simulink model "Day1"  (R2021a)
settings: Solver=VariableStepAuto  StartTime=0.0  StopTime=10.0  RelTol=1e-3
libraries: vexarmcortexlib x2
settings Model: Creator=Kanha  LastModifiedBy=Kanha

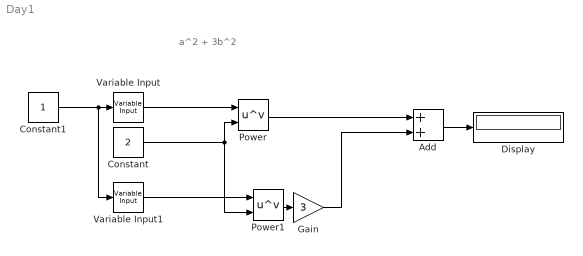
== system Day1 ==
  note: a^2 + 3b^2
  Add : Sum
  Constant : Constant  Value=2
  Constant1 : Constant
  Display : Display
  Gain : Gain  Gain=3
  Power : Math  Operator=pow  SaturateOnIntegerOverflow=on
  Power1 : Math  Operator=pow  SaturateOnIntegerOverflow=on
  Variable Input : vexarmcortexlib/Utilities/Variable Input  low=-127  gain=1  high=127
      settings: SourceProductBaseCode=EC_VEX_MICRO
  Variable Input1 : vexarmcortexlib/Utilities/Variable Input  low=-127  gain=1  high=127
      settings: SourceProductBaseCode=EC_VEX_MICRO
  wires:
  Gain/1 -> Add/2
  Power/1 -> Add/1
  Constant/1 -> Power1/2, Power/2
  Power1/1 -> Gain/1
  Variable Input1/1 -> Power1/1
  Variable Input/1 -> Power/1
  Constant1/1 -> Variable Input1/1, Variable Input/1
  Add/1 -> Display/1
